simulink model "boostObserver"  (R2020a)
settings: Solver=ode45  StartTime=0.0  StopTime=1  FixedStep=0.0005  AbsTol=1e-06  EnableMultiTasking=on
InitFcn:
  | kp=0.01;
  | ki=0.01;
  | 
  | k=2;
  | em=100000000;
  | GE=1/em;
  | GU=k*ki/GE;
  | GCE=k*kp/GU;
model workspace (MAT data in the model file):
  time = 0.8
undefined symbols (not defined in the file): A1, A1aug, A2, b1, B1, B2aug, c, C1, Cmatrix, CvC, deltaA, ie, iLFaultSwitch, iLFaultTime, Kg, Lnew1, Lnew2, LoadAddFactor, LoadRemoveFactor, Lobsmc, P, R, Ro, SourceAddFactor, SourceAddSwitch, SourceRemoveFactor, Ts, VcFaultSwitch, VcFaultTime, ve, Wobsmc, x_e, xe
libraries: PhdLibrary x16, powerlib_meascontrol x2, powerlib x1
settings Model: SimulationMode=accelerator  Creator=d13go  LastModifiedBy=d13go
settings SolverCC: MaxConsecutiveZCs=10000  ZeroCrossAlgorithm=Adaptive  DecoupledContinuousIntegration=on  MinimalZcImpactIntegration=on
settings DataIOCC: SaveFinalState=on  SaveState=on  LoggingToFile=on
settings OptimizationCC: DefaultParameterBehavior=Inlined  UseDivisionForNetSlopeComputation=on  GainParamInheritBuiltInType=on  UseFloatMulNetSlope=on  InlineInvariantSignals=on  EfficientFloat2IntCast=on  LifeSpan=1
settings DebuggingCC: ReadBeforeWriteMsg=DisableAll  WriteAfterWriteMsg=DisableAll  WriteAfterReadMsg=DisableAll  AlgebraicLoopMsg=error  MaxConsecutiveZCsMsg=warning  MaskedZcDiagnostic=none  IgnoredZcDiagnostic=none  MultiTaskDSMMsg=none  SFUnexpectedBacktrackingDiag=warning  SFNoUnconditionalDefaultTransitionDiag=warning  ArithmeticOperatorsInVariantConditions=warning
settings HardwareCC: ProdLongLongMode=on
settings ModelReferenceCC: UpdateModelReferenceTargets=IfOutOfDate
settings SFSimCC: SFSimEcho=off  SimUseLocalCustomCode=off  MATLABDynamicMemAlloc=off  CustomCodeUndefinedFunction=UseInterfaceOnly
settings RTWCC: GenerateReport=on  RTWUseLocalCustomCode=off  LaunchReport=on
settings CodeAppCC: ForceParamTrailComments=on
settings GRTTargetCC: TargetLangStandard=C89/C90 (ANSI)  CombineSignalStateStructs=on  MatFileLogging=off  SupportVariableSizeSignals=on
settings ConfigComp: CovMetricSettings=dw  CovHtmlReporting=on  CovSaveCumulativeToWorkspaceVar=on  CovSaveSingleToWorkspaceVar=on  CovExternalEMLEnable=off
settings SimscapeCC: SimscapeNormalizeSystem=off

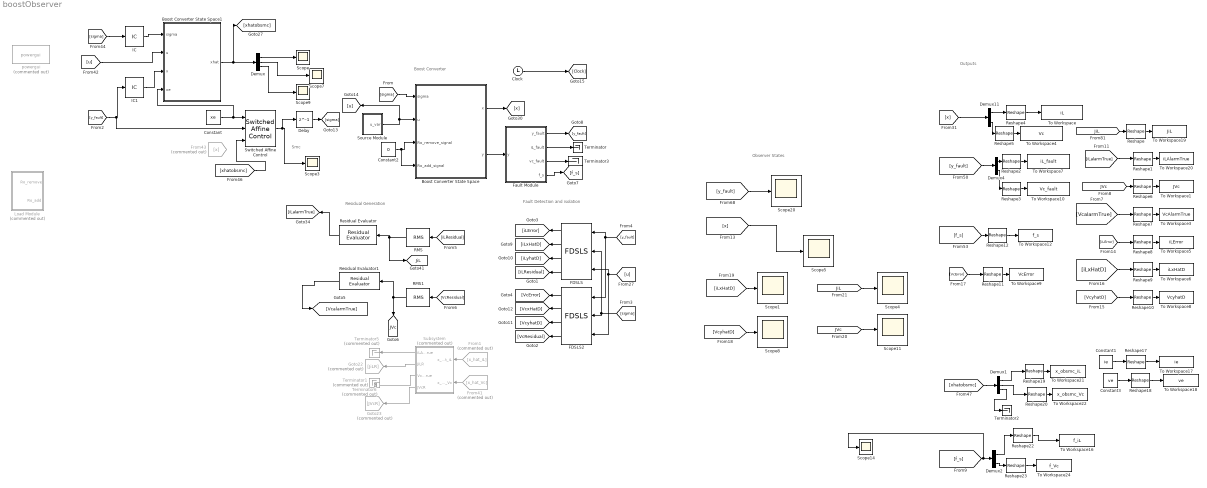
== system boostObserver ==
  note: Smc
  note: Fault Detection and isolation
  note: Outputs
  note: Observer States
  note: Residual Generation
  note: Boost Converter
  Boost Converter State Space : Subsystem  AncestorBlock="PhdLibrary/Boost Converter  State Space"  mask(Boots State-Space model){A1=A1, A2=A2, B1=b1, R=R, Ro=Ro, Cmatrix=C1, c=CvC, LoadAddFactor=LoadAddFactor, LoadRemoveFactor=LoadRemoveFactor}
      mask prompts: A1 "A1 matrix:"; A2 "A2 matrix:"; B1 "B matrix:"; R "Resistance:"; Ro "Output Resistance:"; Cmatrix "Output Matrix:"; c "Capacitance:"; LoadAddFactor "Load add factor:"; LoadRemoveFactor "Load remove factor"
      mask help: Boots State-Space model
      mask Display: disp('Boost')
  Boost Converter State Space1 : Subsystem  mask(Boots State-Space model){A1=A1, A2=A2, B1=B1, R=R, Ro=Ro, Cmatrix=Cmatrix, c=c, LoadAddFactor=LoadAddFactor, LoadRemoveFactor=LoadRemoveFactor}
      mask prompts: A1 "A1 matrix:"; A2 "A2 matrix:"; B1 "B matrix:"; R "Resistance:"; Ro "Output Resistance:"; Cmatrix "Output Matrix:"; c "Capacitance:"; LoadAddFactor "Load add factor:"; LoadRemoveFactor "Load remove factor"
      mask help: Boots State-Space model
      mask Display: disp('Boost')
  Clock : Clock
  Constant : Constant  Value=xe  VectorParams1D=off
  Constant1 : Constant  Value=ie  VectorParams1D=off
  Constant2 : Constant  Value=0
  Constant3 : Constant  Value=ve  VectorParams1D=off
  Delay : Delay  DelayLength=1
  Demux : Demux  Outputs=3
  Demux1 : Demux  Outputs=3
  Demux11 : Demux  Outputs=2
  Demux2 : Demux  Outputs=2
  Demux4 : Demux  Outputs=2
  FDSLS : PhdLibrary/FDSLS  A1=A1  A2=A2  B1=B1  B2=B2  L=Lnew1  yhat0=[0;0]  x0=[0;0]  Qr=[1 0]
      settings: SourceProductName=Phd Diego
  FDSLS2 : PhdLibrary/FDSLS  A1=A1  A2=A2  B1=B1  B2=B2  L=Lnew2  yhat0=[0;0]  x0=[0;0]  Qr=[0 1]
      settings: SourceProductName=Phd Diego
  Fault Module : Subsystem
  From1 : From  Commented=on  GotoTag=x_hat_iL
  From41 : From  Commented=on  GotoTag=x_hat_Vc
  From43 : From  Commented=on  GotoTag=x
  Goto22 : Goto  Commented=on  GotoTag=JiLR
  Goto23 : Goto  Commented=on  GotoTag=JVcR
  IC : InitialCondition
  IC1 : InitialCondition  Value=[0;0]
  Load Module : Subsystem  Commented=on
  RMS : powerlib_meascontrol/Measurements/RMS  TrueRMS=on  Freq=RMSfrequency  RMSInit=0  Ts=Ts
  RMS1 : powerlib_meascontrol/Measurements/RMS  TrueRMS=on  Freq=RMSfrequency  RMSInit=0  Ts=Ts
  Reshape{,1..12,17..20,22..23} (19 alike) : Reshape
  Residual Evaluator : PhdLibrary/Residual Evaluator  Jth=iLJth
      settings: SourceProductName=Phd Diego
  Residual Evaluator1 : PhdLibrary/Residual Evaluator  Jth=VcJth
      settings: SourceProductName=Phd Diego
  Scope{,1,3..5,7..9,11,14,20} (11 alike) : Scope
  Source Module : Subsystem
  Subsystem : Subsystem  Commented=on
  Switched Affine Control : PhdLibrary/Switched Affine Control  A1=A1  A2=A2  B1=b1  B2=b2  P=P
      settings: SourceProductName=Phd Diego
  Terminator : Terminator
  Terminator1 : Terminator  Commented=on
  Terminator2 : Terminator
  Terminator3 : Terminator
  Terminator5 : Terminator  Commented=on
  Terminator6 : Terminator  Commented=on
  To Workspace : ToWorkspace  VariableName=iL  SaveFormat=Timeseries  SampleTime=-1
  To Workspace1 : ToWorkspace  VariableName=JVc  SaveFormat=Timeseries  SampleTime=-1
  To Workspace10 : ToWorkspace  VariableName=Vc_fault  SaveFormat=Timeseries  SampleTime=-1
  To Workspace12 : ToWorkspace  VariableName=f_s  SaveFormat=Timeseries  SampleTime=-1
  To Workspace16 : ToWorkspace  VariableName=f_iL  SaveFormat=Timeseries  SampleTime=-1
  To Workspace17 : ToWorkspace  VariableName=ie  SaveFormat=Timeseries  SampleTime=-1
  To Workspace18 : ToWorkspace  VariableName=ve  SaveFormat=Timeseries  SampleTime=-1
  To Workspace19 : ToWorkspace  VariableName=JiL  SaveFormat=Timeseries  SampleTime=-1
  To Workspace20 : ToWorkspace  VariableName=iLAlarmTrue  SaveFormat=Timeseries  SampleTime=-1
  To Workspace21 : ToWorkspace  VariableName=x_obsmc_iL  SaveFormat=Timeseries  SampleTime=-1
  To Workspace22 : ToWorkspace  VariableName=x_obsmc_Vc  SaveFormat=Timeseries  SampleTime=-1
  To Workspace24 : ToWorkspace  VariableName=f_Vc  SaveFormat=Timeseries  SampleTime=-1
  To Workspace3 : ToWorkspace  VariableName=VcAlarmTrue  SaveFormat=Timeseries  SampleTime=-1
  To Workspace4 : ToWorkspace  VariableName=Vc  SaveFormat=Timeseries  SampleTime=-1
  To Workspace5 : ToWorkspace  VariableName=iLError  SaveFormat=Timeseries  SampleTime=-1
  To Workspace6 : ToWorkspace  VariableName=iLxHatD  SaveFormat=Timeseries  SampleTime=-1
  To Workspace7 : ToWorkspace  VariableName=iL_fault  SaveFormat=Timeseries  SampleTime=-1
  To Workspace8 : ToWorkspace  VariableName=VcyhatD  SaveFormat=Timeseries  SampleTime=-1
  To Workspace9 : ToWorkspace  VariableName=VcError  SaveFormat=Timeseries  SampleTime=-1
  powergui : powerlib/powergui  Priority=1  Commented=on  SimulationMode=Discrete  SampleTime=50e-6  frequency=60  Iterations=50  frequencyindice=0  Pbase=100e6  ErrMax=1e-4  UnitsV=kV  UnitsW=MW  buscounter=0  FunctionMessages=off  echomessages=off  EnableUseOfTLC=off  CurrentSourceSwitches=off  DisableSnubberDevices=off  DisableRonSwitches=off  DisableVfSwitches=off  DisplayEquations=off  AutomaticDiscreteSolvers=off  SolverType=Tustin/Backward Euler (TBE)  Interpol=off  ExternalGateDelay=off  methode=off  Ts=100  x0status=blocks  SPID=on  SwTol=0  HookPort=off  NonlinearTolerance=1e-4  nMaxIteration=100  ContinueOnMaxIteration=off  RestoreLinks=warning  ResistiveCurrentMeasurement=off  Frange=[0:2:500]  Ylog=off  Xlog=on  ShowGrid=off  save=off  variable=ZData  structure=0  ZoomFFT=off  StartTime=0.0  cycles=1  DisplayStyle=1  fundamental=60  FreqAxis=off  MaxFrequency=1000  frequencyindicesteady=1  RmsSteady=1  display=off
  tag scope: JVc=global, JiL=global
  wires:
  Reshape9/1 -> To Workspace6/1
  [y_fault] -> FDSLS2/1, FDSLS/1
  Demux4/1 -> Reshape2/1
  [iLResidual] -> RMS/1
  Clock/1 -> [Clock]
  Boost Converter State Space/1(x) -> [x]
  Fault Module/2(iL_fault) -> Terminator/1
  [JVc] -> Scope11/1
  Demux4/2 -> Reshape3/1
  Reshape7/1 -> To Workspace3/1
  Reshape12/1 -> To Workspace12/1
  Reshape2/1 -> To Workspace7/1
  Residual Evaluator/1 -> [iLalarmTrue]
  Residual Evaluator1/1 -> [VcalarmTrue]
  [y_fault] -> Scope20/1
  [JiL] -> Scope4/1
  [VcyhatD] -> Reshape10/1
  [x] -> Demux11/1
  FDSLS2/2 -> [VcxHatD]
  Constant2/1 -> Boost Converter State Space/4(Ro_add_signal), Boost Converter State Space/3(Ro_remove_signal)
  Source Module/1(u_var) -> [u], Boost Converter State Space/2(u)
  Fault Module/4(f_s) -> [f_s]
  Boost Converter State Space/2(y) -> Fault Module/1(y)
  [VcResidual] -> RMS1/1
  [sigma] -> FDSLS2/2, FDSLS/2
  Demux11/1 -> Reshape4/1
  RMS1/1 -> Residual Evaluator1/1, [JVc]
  RMS/1 -> [JiL], Residual Evaluator/1
  [iLalarmTrue] -> Reshape1/1
  Reshape1/1 -> To Workspace20/1
  [sigma] -> Boost Converter State Space/1(sigma)
  [VcError] -> Reshape11/1
  [x] -> Scope5/1
  FDSLS/4 -> [iLResidual]
  FDSLS2/3 -> [VcyhatD]
  Reshape4/1 -> To Workspace/1
  FDSLS2/1 -> [VcError]
  [VcyhatD] -> Scope8/1
  Reshape11/1 -> To Workspace9/1
  [y_fault] -> Demux4/1
  FDSLS/3 -> [iLyhatD]
  Fault Module/3(vc_fault) -> Terminator3/1
  Reshape8/1 -> To Workspace5/1
  Demux11/2 -> Reshape5/1
  [f_s] -> Reshape12/1
  FDSLS/1 -> [iLError]
  [u] -> FDSLS2/3, FDSLS/3
  [iLError] -> Reshape8/1
  FDSLS2/4 -> [VcResidual]
  Reshape6/1 -> To Workspace1/1
  Fault Module/1(y_fault) -> [y_fault]
  [VcalarmTrue] -> Reshape7/1
  [iLxHatD] -> Reshape9/1
  Reshape3/1 -> To Workspace10/1
  [JiL] -> Reshape/1
  [JVc] -> Reshape6/1
  Reshape/1 -> To Workspace19/1
  Reshape5/1 -> To Workspace4/1
  Reshape10/1 -> To Workspace8/1
  [iLxHatD] -> Scope1/1
  FDSLS/2 -> [iLxHatD]
  Subsystem/1(iLAlarmTrue) -> Terminator5/1
  Subsystem/2(JiLR) -> Goto22/1
  Subsystem/3(VcAlarmTrue) -> Terminator6/1
  Subsystem/4(JVcR) -> Goto23/1
  From1/1 -> Subsystem/1(x_hat_iL)
  From41/1 -> Subsystem/2(x_hat_Vc)
  Constant/1 -> Switched Affine Control/1, Boost Converter State Space1/4(xe)
  Demux/2 -> Scope7/1
  Boost Converter State Space1/1(xhat) -> [xhatobsmc], Demux/1
  Demux/3 -> Scope9/1
  [sigma] -> IC/1
  Demux/1 -> Scope/1
  [u] -> Boost Converter State Space1/2(u)
  IC/1 -> Boost Converter State Space1/1(sigma)
  IC1/1 -> Boost Converter State Space1/3(x)
  [y_fault] -> Switched Affine Control/2, IC1/1
  [xhatobsmc] -> Switched Affine Control/3
  Switched Affine Control/1 -> Delay/1, Scope3/1
  Delay/1 -> [sigma]
  Constant1/1 -> Reshape17/1
  Reshape17/1 -> To Workspace17/1
  Constant3/1 -> Reshape18/1
  Reshape18/1 -> To Workspace18/1
  [xhatobsmc] -> Demux1/1
  Reshape19/1 -> To Workspace21/1
  Demux1/1 -> Reshape19/1
  Reshape20/1 -> To Workspace22/1
  Demux1/2 -> Reshape20/1
  Demux1/3 -> Terminator2/1
  Reshape22/1 -> To Workspace16/1
  Demux2/1 -> Reshape22/1
  Reshape23/1 -> To Workspace24/1
  Demux2/2 -> Reshape23/1
  [f_s] -> Scope14/1, Demux2/1

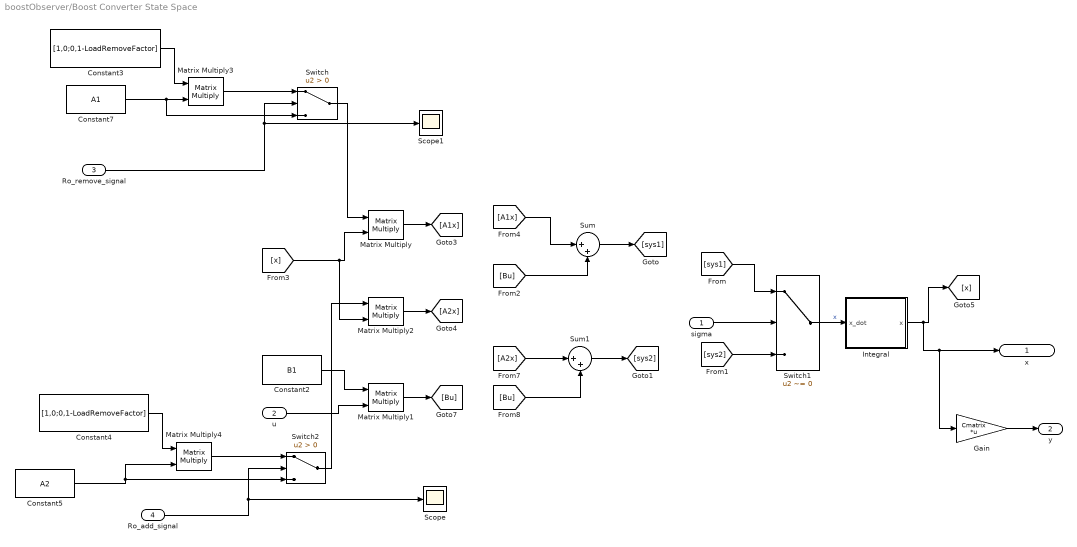
== system boostObserver/Boost Converter State Space ==
  sigma : Inport
  u : Inport  Port=2
  Ro_remove_signal : Inport  Port=3
  Ro_add_signal : Inport  Port=4
  Constant2 : Constant  Value=B1  VectorParams1D=off
  Constant3 : Constant  Value=[1,0;0,1-LoadRemoveFactor]  VectorParams1D=off
  Constant4 : Constant  Value=[1,0;0,1-LoadRemoveFactor]  VectorParams1D=off
  Constant5 : Constant  Value=A2  VectorParams1D=off
  Constant7 : Constant  Value=A1  VectorParams1D=off
  Gain : Gain  Gain=Cmatrix  Multiplication=Matrix(K*u)
  Integral : Subsystem
  Matrix Multiply{,1..4} (5 alike) : Product  Multiplication=Matrix(*)
  Scope : Scope
  Scope1 : Scope
  Sum : Sum  Inputs=|++
  Sum1 : Sum  Inputs=|++
  Switch : Switch  Criteria=u2 > Threshold
  Switch1 : Switch  Criteria=u2 ~= 0
  Switch2 : Switch  Criteria=u2 > Threshold
  x : Outport
  y : Outport  Port=2
  wires:
  Switch2/1 -> Matrix Multiply2/1
  Ro_add_signal/1 -> Scope/1, Switch2/2
  Constant5/1 -> Matrix Multiply4/2, Switch2/3
  Matrix Multiply4/1 -> Switch2/1
  Constant4/1 -> Matrix Multiply4/1
  Switch/1 -> Matrix Multiply/1
  Ro_remove_signal/1 -> Scope1/1, Switch/2
  Matrix Multiply3/1 -> Switch/1
  Constant7/1 -> Switch/3, Matrix Multiply3/2
  Constant3/1 -> Matrix Multiply3/1
  Gain/1 -> y/1
  Integral/1(x) -> [x], x/1, Gain/1
  u/1 -> Matrix Multiply1/2
  Matrix Multiply1/1 -> [Bu]
  Constant2/1 -> Matrix Multiply1/1
  sigma/1 -> Switch1/2
  [A2x] -> Sum1/1
  Switch1/1 -> Integral/1(x_dot)  "x"
  Sum1/1 -> [sys2]
  Sum/1 -> [sys1]
  Matrix Multiply/1 -> [A1x]
  Matrix Multiply2/1 -> [A2x]
  [Bu] -> Sum/2
  [Bu] -> Sum1/2
  [x] -> Matrix Multiply/2, Matrix Multiply2/2
  [A1x] -> Sum/1
  [sys1] -> Switch1/1
  [sys2] -> Switch1/3

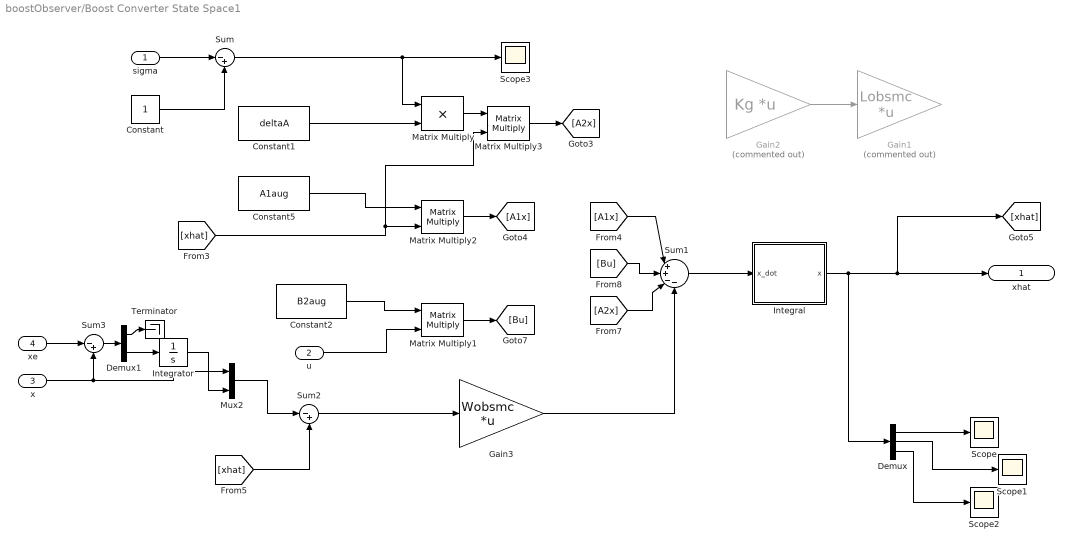
== system boostObserver/Boost Converter State Space1 ==
  sigma : Inport
  u : Inport  Port=2
  x : Inport  Port=3
  xe : Inport  Port=4
  Constant : Constant
  Constant1 : Constant  Value=deltaA  VectorParams1D=off
  Constant2 : Constant  Value=B2aug  VectorParams1D=off
  Constant5 : Constant  Value=A1aug  VectorParams1D=off
  Demux : Demux  Outputs=3
  Demux1 : Demux  Outputs=2
  Gain1 : Gain  Commented=on  Gain=Lobsmc  Multiplication=Matrix(K*u)
  Gain2 : Gain  Commented=on  Gain=Kg  Multiplication=Matrix(K*u)
  Gain3 : Gain  Gain=Wobsmc  Multiplication=Matrix(K*u)
  Integral : Subsystem
  Integrator : Integrator
  Matrix Multiply : Product
  Matrix Multiply1 : Product  Multiplication=Matrix(*)
  Matrix Multiply2 : Product  Multiplication=Matrix(*)
  Matrix Multiply3 : Product  Multiplication=Matrix(*)
  Mux2 : Mux  Inputs=2
  Scope{,1..3} (4 alike) : Scope
  Sum : Sum  Inputs=|-+
  Sum1 : Sum  Inputs=|++--
  Sum2 : Sum  Inputs=|-+
  Sum3 : Sum  Inputs=|-+
  Terminator : Terminator
  xhat : Outport
  wires:
  u/1 -> Matrix Multiply1/2
  Matrix Multiply1/1 -> [Bu]
  Constant2/1 -> Matrix Multiply1/1
  Matrix Multiply2/1 -> [A1x]
  [Bu] -> Sum1/2
  [xhat] -> Matrix Multiply3/2, Matrix Multiply2/2
  [xhat] -> Sum2/2
  Demux/2 -> Scope1/1
  Integral/1(x) -> [xhat], xhat/1, Demux/1
  Demux/1 -> Scope/1
  Demux/3 -> Scope2/1
  Gain2/1 -> Gain1/1
  Constant5/1 -> Matrix Multiply2/1
  Sum1/1 -> Integral/1(x_dot)
  Constant1/1 -> Matrix Multiply/2
  Matrix Multiply/1 -> Matrix Multiply3/1
  Matrix Multiply3/1 -> [A2x]
  sigma/1 -> Sum/1
  Sum/1 -> Scope3/1, Matrix Multiply/1
  Constant/1 -> Sum/2
  Sum2/1 -> Gain3/1
  xe/1 -> Sum3/1
  x/1 -> Mux2/1, Sum3/2
  Sum3/1 -> Demux1/1
  Demux1/2 -> Integrator/1
  Integrator/1 -> Mux2/2
  Demux1/1 -> Terminator/1
  Mux2/1 -> Sum2/1
  [A1x] -> Sum1/1
  [A2x] -> Sum1/3
  Gain3/1 -> Sum1/4

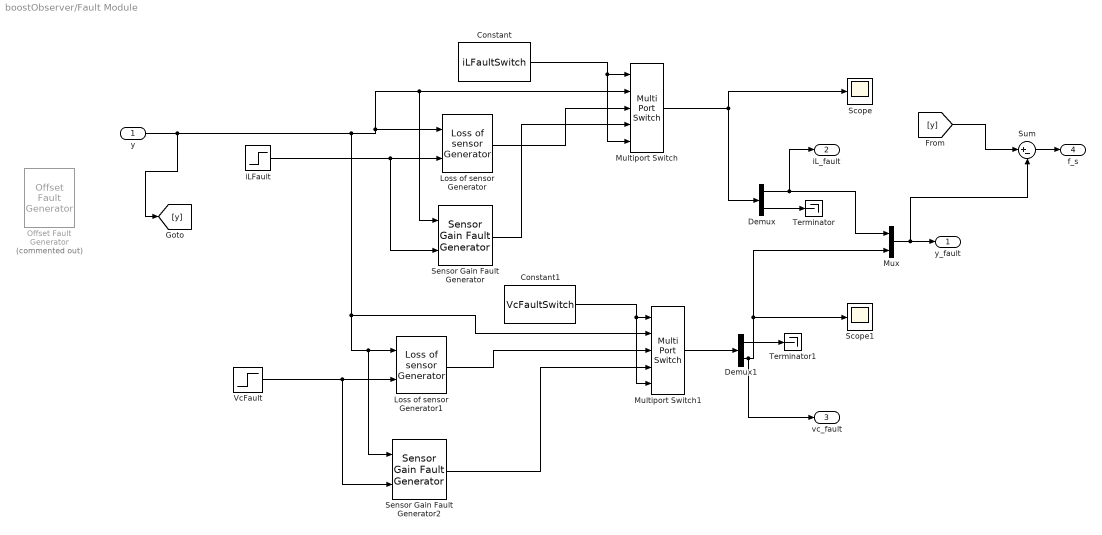
== system boostObserver/Fault Module ==
  y : Inport
  Constant : Constant  Value=iLFaultSwitch
  Constant1 : Constant  Value=VcFaultSwitch
  Demux : Demux  Outputs=2
  Demux1 : Demux  Outputs=2
  Loss of sensor Generator : PhdLibrary/Loss of sensor Generator
      settings: SourceProductName=Phd Diego
  Loss of sensor Generator1 : PhdLibrary/Loss of sensor Generator
      settings: SourceProductName=Phd Diego
  Multiport Switch : MultiPortSwitch  DataPortOrder=Zero-based contiguous  DataPortForDefault=Additional data port  zeroidx=on
  Multiport Switch1 : MultiPortSwitch  DataPortOrder=Zero-based contiguous  DataPortForDefault=Additional data port  zeroidx=on
  Mux : Mux  Inputs=2
  Offset Fault Generator : PhdLibrary/Offset Fault Generator  Commented=on  s1gain=20  s2gain=20
      settings: SourceProductName=Phd Diego
  Scope : Scope
  Scope1 : Scope
  Sensor Gain Fault Generator : PhdLibrary/Sensor Gain Fault Generator  s1gain=iLGainFaultFactor  s2gain=VcGainFaultFactor
      settings: SourceProductName=Phd Diego
  Sensor Gain Fault Generator2 : PhdLibrary/Sensor Gain Fault Generator  s1gain=iLGainFaultFactor  s2gain=VcGainFaultFactor
      settings: SourceProductName=Phd Diego
  Sum : Sum  Inputs=|+-
  Terminator : Terminator
  Terminator1 : Terminator
  VcFault : Step  Time=VcFaultTime  After=2  SampleTime=0
  iLFault : Step  Time=iLFaultTime  SampleTime=0
  y_fault : Outport
  iL_fault : Outport  Port=2
  vc_fault : Outport  Port=3
  f_s : Outport  Port=4
  wires:
  iLFault/1 -> Sensor Gain Fault Generator/2, Loss of sensor Generator/2
  y/1 -> [y], Multiport Switch1/2, Sensor Gain Fault Generator2/1, Loss of sensor Generator1/1, Sensor Gain Fault Generator/1, Multiport Switch/2, Loss of sensor Generator/1
  VcFault/1 -> Sensor Gain Fault Generator2/2, Loss of sensor Generator1/2
  Constant/1 -> Multiport Switch/5, Multiport Switch/1
  Constant1/1 -> Multiport Switch1/5, Multiport Switch1/1
  Multiport Switch/1 -> Demux/1, Scope/1
  Multiport Switch1/1 -> Demux1/1
  Demux/2 -> Terminator/1
  Demux/1 -> iL_fault/1, Mux/1
  Mux/1 -> Sum/2, y_fault/1
  Demux1/1 -> Terminator1/1
  Demux1/2 -> vc_fault/1, Mux/2, Scope1/1
  Loss of sensor Generator/1 -> Multiport Switch/3
  Sensor Gain Fault Generator/1 -> Multiport Switch/4
  Sensor Gain Fault Generator2/1 -> Multiport Switch1/4
  Loss of sensor Generator1/1 -> Multiport Switch1/3
  [y] -> Sum/1
  Sum/1 -> f_s/1

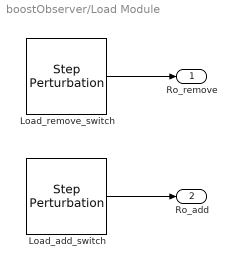
== system boostObserver/Load Module ==
  Load_add_switch : PhdLibrary/Step Perturbation  SignalSwitch=LoadAddSignalSwitch  InitialMagnitude=0  InitialTime=LoadAddTime  Magnitude=1  Duration=LoadAddDuration  enabled=LoadAddSwitch
      settings: SourceProductName=Phd Diego
  Load_remove_switch : PhdLibrary/Step Perturbation  SignalSwitch=LoadRemoveSignalSwitch  InitialMagnitude=0  InitialTime=LoadRemoveTime  Magnitude=1  Duration=LoadRemoveDuration  enabled=LoadRemoveSwitch
      settings: SourceProductName=Phd Diego
  Ro_remove : Outport
  Ro_add : Outport  Port=2
  wires:
  Load_remove_switch/1 -> Ro_remove/1
  Load_add_switch/1 -> Ro_add/1

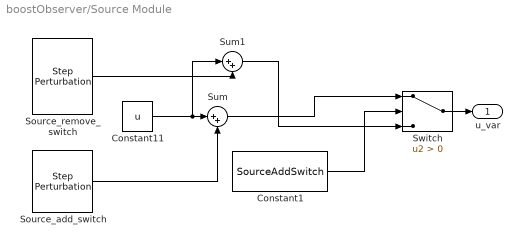
== system boostObserver/Source Module ==
  Constant1 : Constant  Value=SourceAddSwitch  VectorParams1D=off
  Constant11 : Constant  Value=u
  Source_add_switch : PhdLibrary/Step Perturbation  SignalSwitch=SourceAddSignalSwitch  InitialMagnitude=0  InitialTime=SourceAddTime  Magnitude=SourceAddFactor*u  Duration=SourceAddDuration  enabled=SourceAddSwitch
      settings: SourceProductName=Phd Diego
  Source_remove_switch : PhdLibrary/Step Perturbation  SignalSwitch=SourceRemoveSignalSwitch  InitialMagnitude=0  InitialTime=SourceRemoveTime  Magnitude=-SourceRemoveFactor*u  Duration=SourceRemoveDuration  enabled=SourceRemoveSwitch
      settings: SourceProductName=Phd Diego
  Sum : Sum  Inputs=|++
  Sum1 : Sum  Inputs=|++
  Switch : Switch  Criteria=u2 > Threshold
  u_var : Outport
  wires:
  Sum1/1 -> Switch/3
  Sum/1 -> Switch/1
  Constant11/1 -> Sum1/1, Sum/1
  Switch/1 -> u_var/1
  Source_add_switch/1 -> Sum/2
  Source_remove_switch/1 -> Sum1/2
  Constant1/1 -> Switch/2

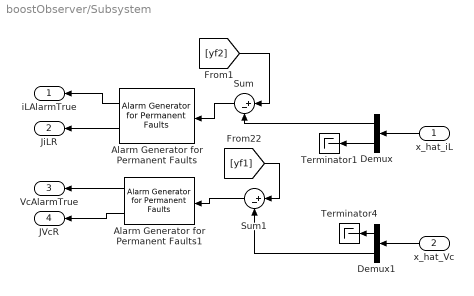
== system boostObserver/Subsystem ==
  x_hat_iL : Inport
  x_hat_Vc : Inport  Port=2
  Alarm Generator for Permanent Faults : PhdLibrary/Alarm Generator for Permanent Faults  Jth=0  r0=0
      settings: SourceProductName=Phd Diego
  Alarm Generator for Permanent Faults1 : PhdLibrary/Alarm Generator for Permanent Faults  Jth=0  r0=0
      settings: SourceProductName=Phd Diego
  Demux : Demux  Outputs=2
  Demux1 : Demux  Outputs=2
  Sum : Sum  Inputs=|+-
  Sum1 : Sum  Inputs=|+-
  Terminator1 : Terminator
  Terminator4 : Terminator
  iLAlarmTrue : Outport
  JiLR : Outport  Port=2
  VcAlarmTrue : Outport  Port=3
  JVcR : Outport  Port=4
  wires:
  [yf1] -> Sum1/1
  Alarm Generator for Permanent Faults1/2 -> JVcR/1
  [yf2] -> Sum/1
  Sum1/1 -> Alarm Generator for Permanent Faults1/1
  Sum/1 -> Alarm Generator for Permanent Faults/1
  Alarm Generator for Permanent Faults/2 -> JiLR/1
  Alarm Generator for Permanent Faults/1 -> iLAlarmTrue/1
  Alarm Generator for Permanent Faults1/1 -> VcAlarmTrue/1
  Demux/2 -> Terminator1/1
  Demux/1 -> Sum/2
  x_hat_iL/1 -> Demux/1
  Demux1/1 -> Terminator4/1
  Demux1/2 -> Sum1/2
  x_hat_Vc/1 -> Demux1/1

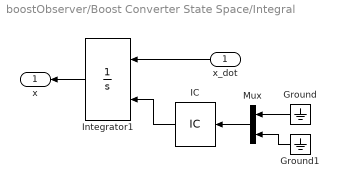
== system boostObserver/Boost Converter State Space/Integral ==
  x_dot : Inport
  Ground : Ground
  Ground1 : Ground
  IC : InitialCondition  Value=[0;0]
  Integrator1 : Integrator  InitialConditionSource=external  InitialCondition=[-x_e; 0; 0]
  Mux : Mux  Inputs=2
  x : Outport
  wires:
  Mux/1 -> IC/1
  Ground/1 -> Mux/1
  Ground1/1 -> Mux/2
  IC/1 -> Integrator1/2
  Integrator1/1 -> x/1
  x_dot/1 -> Integrator1/1

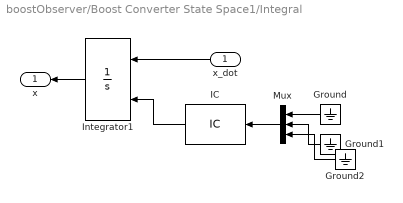
== system boostObserver/Boost Converter State Space1/Integral ==
  x_dot : Inport
  Ground : Ground
  Ground1 : Ground
  Ground2 : Ground
  IC : InitialCondition  Value=[0;0;0]
  Integrator1 : Integrator  InitialConditionSource=external  InitialCondition=[-x_e; 0; 0]
  Mux : Mux  Inputs=3
  x : Outport
  wires:
  Mux/1 -> IC/1
  Ground/1 -> Mux/1
  Ground1/1 -> Mux/2
  IC/1 -> Integrator1/2
  Integrator1/1 -> x/1
  x_dot/1 -> Integrator1/1
  Ground2/1 -> Mux/3
